simulink model "robot"  (R2018a)
settings: Solver=VariableStepAuto  StartTime=0.0  StopTime=10  RelTol=1e-3
undefined symbols (not defined in the file or in its folder): arm, belt, bread1, bread2
settings Model: Creator=hugo  LastModifiedBy=hugo

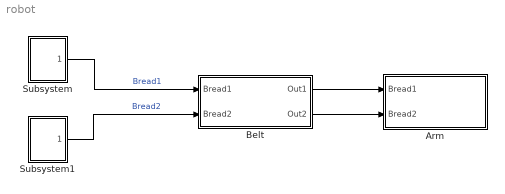
== system robot ==
  Arm : Subsystem
  Belt : Subsystem
  Subsystem : Subsystem
  Subsystem1 : Subsystem
  wires:
  Subsystem/1(Bread1) -> Belt/1(Bread1)  "Bread1"
  Subsystem1/1(Bread2) -> Belt/2(Bread2)  "Bread2"
  Belt/1(Out1) -> Arm/1(Bread1)
  Belt/2(Out2) -> Arm/2(Bread2)

== system robot/Arm ==
  Bread1 : Inport
  Bread2 : Inport  Port=2
  Home Position : Subsystem
  Laser Scanner : Subsystem
  Laser Scanner1 : Subsystem
  MoveArmToBread1 : Subsystem
  MoveArmToBread2 : Subsystem
  MoveArmToHome : Subsystem
  Terminator : Terminator
  To Workspace : ToWorkspace  VariableName=bread1SIM  SaveFormat=Timeseries  SampleTime=-1
  wires:
  Bread1/1 -> To Workspace/1, Laser Scanner/1(In1)
  MoveArmToBread1/1(endEffector) -> MoveArmToBread2/1(Starting Position)
  MoveArmToBread2/1(endEffector) -> MoveArmToHome/1(Starting Position)
  Home Position/1(Home) -> MoveArmToHome/2(Final Position), MoveArmToBread1/1(Starting Position)
  MoveArmToHome/1(endEffector) -> Terminator/1
  Laser Scanner/1(Out1) -> MoveArmToBread1/2(Final Position)
  Bread2/1 -> Laser Scanner1/1(In1)
  Laser Scanner1/1(Out1) -> MoveArmToBread2/2(Final Position)

== system robot/Belt ==
  Bread1 : Inport
  Bread2 : Inport  Port=2
  Constant : Constant  Value=belt.speed
  Movement1 : Subsystem
  Movement2 : Subsystem
  Out1 : Outport
  Out2 : Outport  Port=2
  wires:
  Bread1/1 -> Movement2/2(Bread)
  Movement2/1(Out2) -> Out1/1  "Bread1"
  Movement1/1(Out2) -> Out2/1  "Bread2"
  Bread2/1 -> Movement1/2(Bread)
  Constant/1 -> Movement1/1(Speed), Movement2/1(Speed)

== system robot/Subsystem ==
  Constant : Constant  Value=bread1.x
  Constant1 : Constant  Value=bread1.y
  Constant2 : Constant  Value=bread1.z
  Constant3 : Constant  Value=bread1.theta
  Mux : Mux
  Bread1 : Outport
  wires:
  Mux/1 -> Bread1/1
  Constant/1 -> Mux/1
  Constant1/1 -> Mux/2
  Constant2/1 -> Mux/3
  Constant3/1 -> Mux/4

== system robot/Subsystem1 ==
  Constant : Constant  Value=bread2.x
  Constant1 : Constant  Value=bread2.y
  Constant2 : Constant  Value=bread2.z
  Constant3 : Constant  Value=bread2.theta
  Mux : Mux
  Bread2 : Outport
  wires:
  Mux/1 -> Bread2/1
  Constant/1 -> Mux/1
  Constant1/1 -> Mux/2
  Constant2/1 -> Mux/3
  Constant3/1 -> Mux/4

== system robot/Arm/Home Position ==
  Constant : Constant  Value=arm.homeX
  Constant1 : Constant  Value=arm.homeZ
  Constant2 : Constant  Value=arm.homeY
  Constant3 : Constant  Value=arm.homeZ
  Mux : Mux
  Home : Outport
  wires:
  Constant1/1 -> Mux/3
  Constant2/1 -> Mux/2
  Constant/1 -> Mux/1
  Mux/1 -> Home/1
  Constant3/1 -> Mux/4

== system robot/Arm/Laser Scanner ==
  In1 : Inport
  Demux : Demux
  Mux : Mux
  Switch : Switch  Threshold=0.28
  Out1 : Outport
  wires:
  Switch/1 -> Mux/2
  Demux/4 -> Mux/4  "theta"
  Demux/2 -> Switch/1, Switch/3, Switch/2  "y"
  Demux/1 -> Mux/1  "x"
  Demux/3 -> Mux/3  "z"
  In1/1 -> Demux/1
  Mux/1 -> Out1/1

== system robot/Arm/Laser Scanner1 ==
  In1 : Inport
  Demux : Demux
  Mux : Mux
  Switch : Switch  Threshold=0.28
  Out1 : Outport
  wires:
  Switch/1 -> Mux/2
  Demux/4 -> Mux/4  "theta"
  Demux/2 -> Switch/1, Switch/3, Switch/2  "y"
  Demux/1 -> Mux/1  "x"
  Demux/3 -> Mux/3  "z"
  In1/1 -> Demux/1
  Mux/1 -> Out1/1

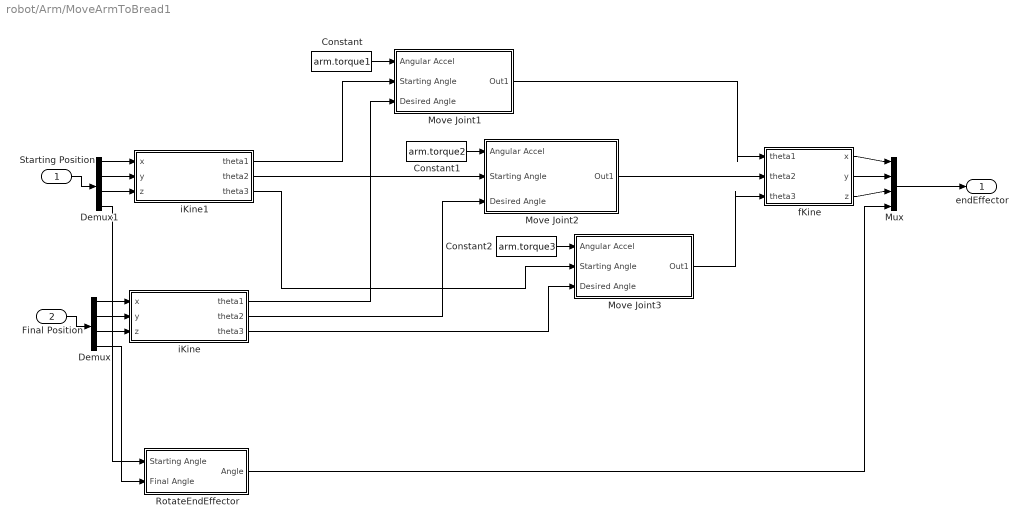
== system robot/Arm/MoveArmToBread1 ==
  Starting Position : Inport
  Final Position : Inport  Port=2
  Constant : Constant  Value=arm.torque1
  Constant1 : Constant  Value=arm.torque2
  Constant2 : Constant  Value=arm.torque3
  Demux : Demux
  Demux1 : Demux
  Move Joint1 : Subsystem
  Move Joint2 : Subsystem
  Move Joint3 : Subsystem
  Mux : Mux
  RotateEndEffector : Subsystem
  fKine : MATLAB Function  TreatAsAtomicUnit=on
  iKine : MATLAB Function  TreatAsAtomicUnit=on
  iKine1 : MATLAB Function  TreatAsAtomicUnit=on
  endEffector : Outport
  wires:
  iKine/1(theta1) -> Move Joint1/3(Desired Angle)
  Starting Position/1 -> Demux1/1
  Demux/2 -> iKine/2(y)
  Demux/3 -> iKine/3(z)
  iKine/2(theta2) -> Move Joint2/3(Desired Angle)
  iKine/3(theta3) -> Move Joint3/3(Desired Angle)
  Move Joint2/1(Out1) -> fKine/2(theta2)
  Move Joint3/1(Out1) -> fKine/3(theta3)
  fKine/1(x) -> Mux/1
  fKine/2(y) -> Mux/2
  fKine/3(z) -> Mux/3
  Mux/1 -> endEffector/1
  Move Joint1/1(Out1) -> fKine/1(theta1)
  Final Position/1 -> Demux/1
  Demux/1 -> iKine/1(x)
  Demux1/2 -> iKine1/2(y)
  Demux1/1 -> iKine1/1(x)
  Demux1/3 -> iKine1/3(z)
  iKine1/1(theta1) -> Move Joint1/2(Starting Angle)
  iKine1/2(theta2) -> Move Joint2/2(Starting Angle)
  iKine1/3(theta3) -> Move Joint3/2(Starting Angle)
  Constant2/1 -> Move Joint3/1(Angular Accel)
  Constant1/1 -> Move Joint2/1(Angular Accel)
  Constant/1 -> Move Joint1/1(Angular Accel)
  Demux1/4 -> RotateEndEffector/1(Starting Angle)
  Demux/4 -> RotateEndEffector/2(Final Angle)
  RotateEndEffector/1(Angle) -> Mux/4

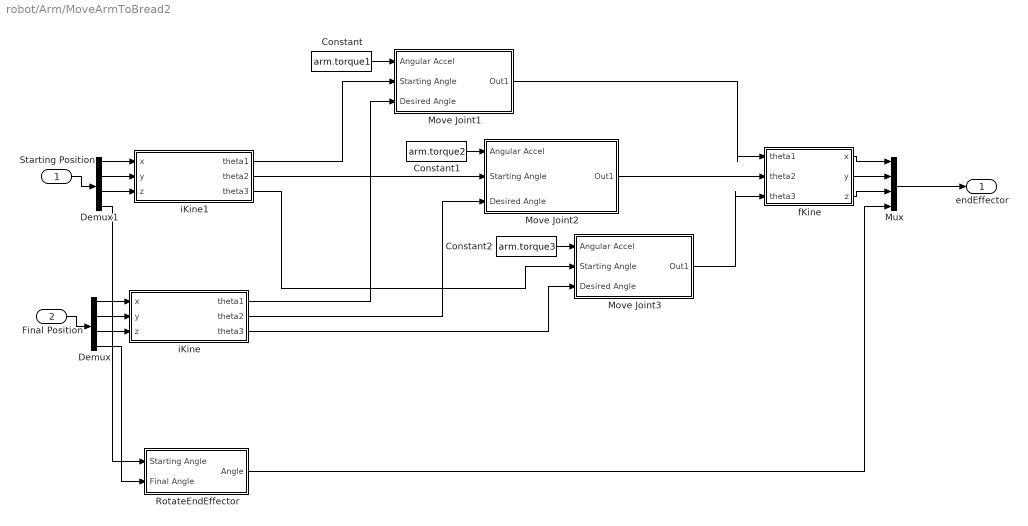
== system robot/Arm/MoveArmToBread2 ==
  Starting Position : Inport
  Final Position : Inport  Port=2
  Constant : Constant  Value=arm.torque1
  Constant1 : Constant  Value=arm.torque2
  Constant2 : Constant  Value=arm.torque3
  Demux : Demux
  Demux1 : Demux
  Move Joint1 : Subsystem
  Move Joint2 : Subsystem
  Move Joint3 : Subsystem
  Mux : Mux
  RotateEndEffector : Subsystem
  fKine : MATLAB Function  TreatAsAtomicUnit=on
  iKine : MATLAB Function  TreatAsAtomicUnit=on
  iKine1 : MATLAB Function  TreatAsAtomicUnit=on
  endEffector : Outport
  wires:
  iKine/1(theta1) -> Move Joint1/3(Desired Angle)
  Starting Position/1 -> Demux1/1
  Demux/2 -> iKine/2(y)
  Demux/3 -> iKine/3(z)
  iKine/2(theta2) -> Move Joint2/3(Desired Angle)
  iKine/3(theta3) -> Move Joint3/3(Desired Angle)
  Move Joint2/1(Out1) -> fKine/2(theta2)
  Move Joint3/1(Out1) -> fKine/3(theta3)
  fKine/1(x) -> Mux/1
  fKine/2(y) -> Mux/2
  fKine/3(z) -> Mux/3
  Mux/1 -> endEffector/1
  Move Joint1/1(Out1) -> fKine/1(theta1)
  Final Position/1 -> Demux/1
  Demux/1 -> iKine/1(x)
  Demux1/2 -> iKine1/2(y)
  Demux1/1 -> iKine1/1(x)
  Demux1/3 -> iKine1/3(z)
  iKine1/1(theta1) -> Move Joint1/2(Starting Angle)
  iKine1/2(theta2) -> Move Joint2/2(Starting Angle)
  iKine1/3(theta3) -> Move Joint3/2(Starting Angle)
  Constant2/1 -> Move Joint3/1(Angular Accel)
  Constant1/1 -> Move Joint2/1(Angular Accel)
  Constant/1 -> Move Joint1/1(Angular Accel)
  Demux1/4 -> RotateEndEffector/1(Starting Angle)
  Demux/4 -> RotateEndEffector/2(Final Angle)
  RotateEndEffector/1(Angle) -> Mux/4

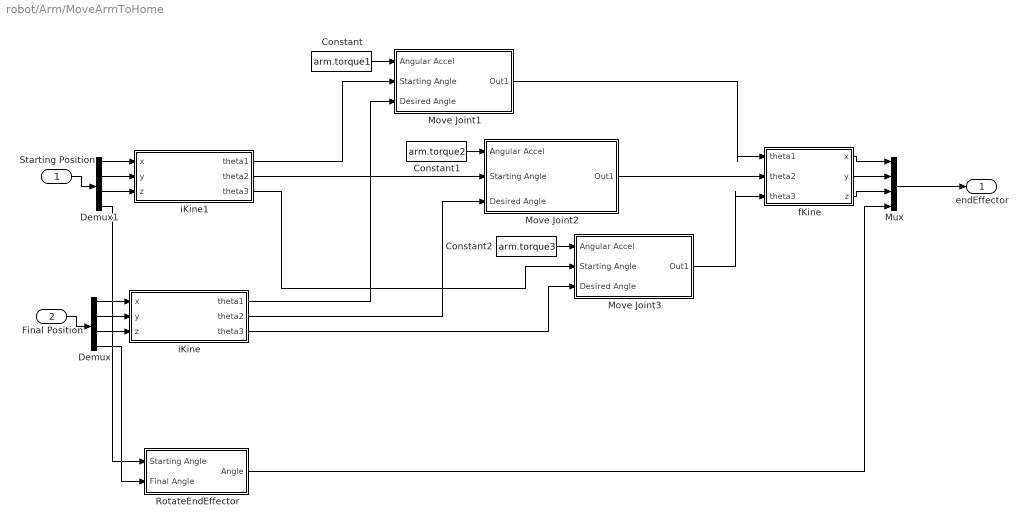
== system robot/Arm/MoveArmToHome ==
  Starting Position : Inport
  Final Position : Inport  Port=2
  Constant : Constant  Value=arm.torque1
  Constant1 : Constant  Value=arm.torque2
  Constant2 : Constant  Value=arm.torque3
  Demux : Demux
  Demux1 : Demux
  Move Joint1 : Subsystem
  Move Joint2 : Subsystem
  Move Joint3 : Subsystem
  Mux : Mux
  RotateEndEffector : Subsystem
  fKine : MATLAB Function  TreatAsAtomicUnit=on
  iKine : MATLAB Function  TreatAsAtomicUnit=on
  iKine1 : MATLAB Function  TreatAsAtomicUnit=on
  endEffector : Outport
  wires:
  iKine/1(theta1) -> Move Joint1/3(Desired Angle)
  Starting Position/1 -> Demux1/1
  Demux/2 -> iKine/2(y)
  Demux/3 -> iKine/3(z)
  iKine/2(theta2) -> Move Joint2/3(Desired Angle)
  iKine/3(theta3) -> Move Joint3/3(Desired Angle)
  Move Joint2/1(Out1) -> fKine/2(theta2)
  Move Joint3/1(Out1) -> fKine/3(theta3)
  fKine/1(x) -> Mux/1
  fKine/2(y) -> Mux/2
  fKine/3(z) -> Mux/3
  Mux/1 -> endEffector/1
  Move Joint1/1(Out1) -> fKine/1(theta1)
  Final Position/1 -> Demux/1
  Demux/1 -> iKine/1(x)
  Demux1/2 -> iKine1/2(y)
  Demux1/1 -> iKine1/1(x)
  Demux1/3 -> iKine1/3(z)
  iKine1/1(theta1) -> Move Joint1/2(Starting Angle)
  iKine1/2(theta2) -> Move Joint2/2(Starting Angle)
  iKine1/3(theta3) -> Move Joint3/2(Starting Angle)
  Constant2/1 -> Move Joint3/1(Angular Accel)
  Constant1/1 -> Move Joint2/1(Angular Accel)
  Constant/1 -> Move Joint1/1(Angular Accel)
  Demux1/4 -> RotateEndEffector/1(Starting Angle)
  Demux/4 -> RotateEndEffector/2(Final Angle)
  RotateEndEffector/1(Angle) -> Mux/4

== system robot/Belt/Movement1 ==
  Speed : Inport
  Bread : Inport  Port=2
  Demux : Demux
  Integrator : Integrator
  Mux : Mux
  Sum : Sum  Inputs=|++
  Out2 : Outport
  wires:
  Bread/1 -> Demux/1  "bread"
  Demux/1 -> Mux/1  "x"
  Demux/3 -> Mux/3  "z"
  Demux/2 -> Sum/2  "y"
  Mux/1 -> Out2/1  "bread.moving"
  Sum/1 -> Mux/2  "y"
  Demux/4 -> Mux/4  "theta"
  Speed/1 -> Integrator/1
  Integrator/1 -> Sum/1

== system robot/Belt/Movement2 ==
  Speed : Inport
  Bread : Inport  Port=2
  Demux : Demux
  Integrator : Integrator
  Mux : Mux
  Sum : Sum  Inputs=|+-
  Out2 : Outport
  wires:
  Bread/1 -> Demux/1  "bread"
  Demux/1 -> Mux/1  "x"
  Demux/3 -> Mux/3  "z"
  Mux/1 -> Out2/1  "bread.moving"
  Sum/1 -> Mux/2  "y"
  Demux/4 -> Mux/4  "theta"
  Speed/1 -> Integrator/1
  Demux/2 -> Sum/1  "y"
  Integrator/1 -> Sum/2

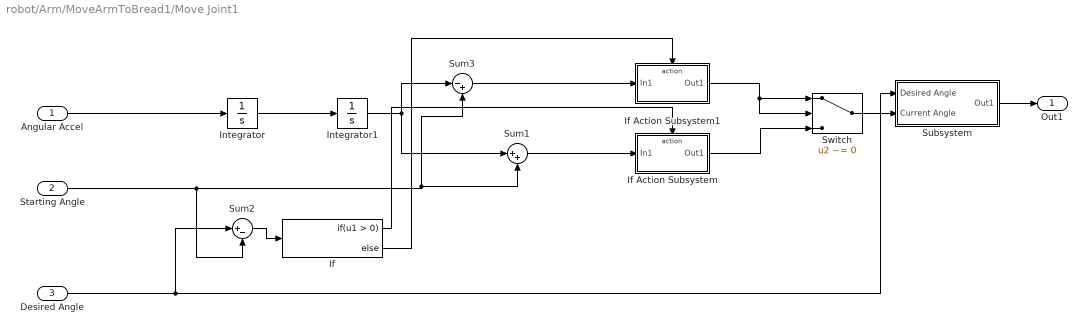
== system robot/Arm/MoveArmToBread1/Move Joint1 ==
  Angular Accel : Inport
  Starting Angle : Inport  Port=2
  Desired Angle : Inport  Port=3
  If : If
  If Action Subsystem : Subsystem  TreatAsAtomicUnit=on
  If Action Subsystem1 : Subsystem  TreatAsAtomicUnit=on
  Integrator : Integrator
  Integrator1 : Integrator
  Subsystem : Subsystem
  Sum1 : Sum  Inputs=|++
  Sum2 : Sum  Inputs=|+-
  Sum3 : Sum  Inputs=|-+
  Switch : Switch  Criteria=u2 ~= 0
  Out1 : Outport
  wires:
  Angular Accel/1 -> Integrator/1
  Integrator/1 -> Integrator1/1
  If Action Subsystem/1(Out1) -> Switch/3
  Sum2/1 -> If/1
  If/2 -> If Action Subsystem1/Action
  Starting Angle/1 -> Sum2/2, Sum3/2, Sum1/2
  Desired Angle/1 -> Subsystem/1(Desired Angle), Sum2/1
  If Action Subsystem1/1(Out1) -> Switch/1, Switch/2
  If/1 -> If Action Subsystem/Action
  Integrator1/1 -> Sum1/1, Sum3/1
  Sum3/1 -> If Action Subsystem1/1(In1)
  Sum1/1 -> If Action Subsystem/1(In1)
  Switch/1 -> Subsystem/2(Current Angle)
  Subsystem/1(Out1) -> Out1/1

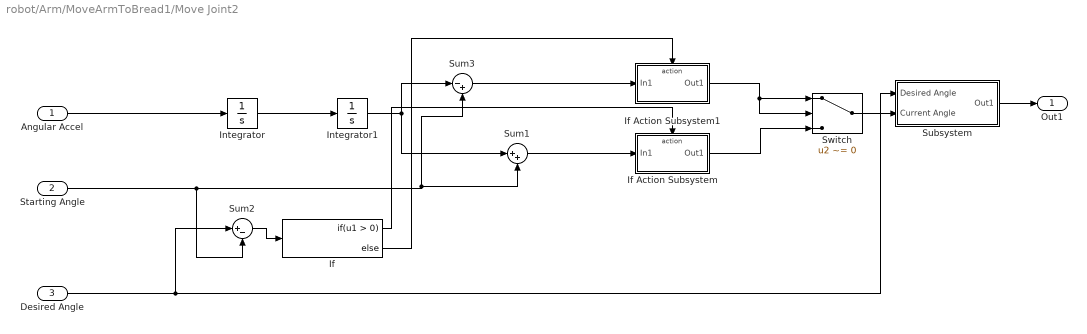
== system robot/Arm/MoveArmToBread1/Move Joint2 ==
  Angular Accel : Inport
  Starting Angle : Inport  Port=2
  Desired Angle : Inport  Port=3
  If : If
  If Action Subsystem : Subsystem  TreatAsAtomicUnit=on
  If Action Subsystem1 : Subsystem  TreatAsAtomicUnit=on
  Integrator : Integrator
  Integrator1 : Integrator
  Subsystem : Subsystem
  Sum1 : Sum  Inputs=|++
  Sum2 : Sum  Inputs=|+-
  Sum3 : Sum  Inputs=|-+
  Switch : Switch  Criteria=u2 ~= 0
  Out1 : Outport
  wires:
  Angular Accel/1 -> Integrator/1
  Integrator/1 -> Integrator1/1
  If Action Subsystem/1(Out1) -> Switch/3
  Sum2/1 -> If/1
  If/2 -> If Action Subsystem1/Action
  Starting Angle/1 -> Sum2/2, Sum3/2, Sum1/2
  Desired Angle/1 -> Subsystem/1(Desired Angle), Sum2/1
  If Action Subsystem1/1(Out1) -> Switch/1, Switch/2
  If/1 -> If Action Subsystem/Action
  Integrator1/1 -> Sum1/1, Sum3/1
  Sum3/1 -> If Action Subsystem1/1(In1)
  Sum1/1 -> If Action Subsystem/1(In1)
  Switch/1 -> Subsystem/2(Current Angle)
  Subsystem/1(Out1) -> Out1/1

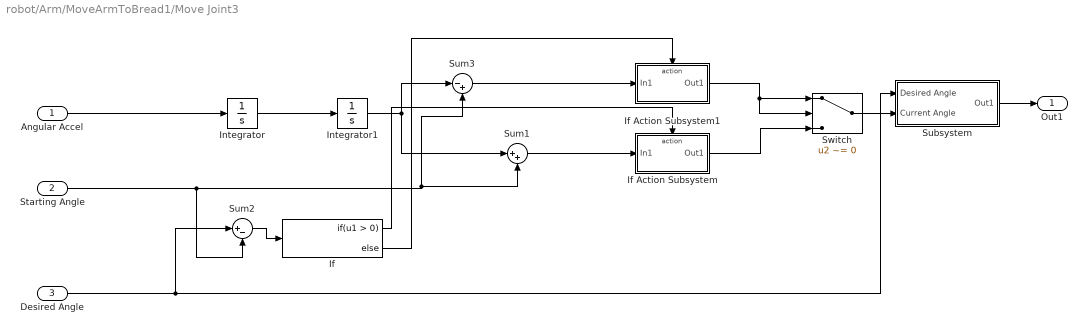
== system robot/Arm/MoveArmToBread1/Move Joint3 ==
  Angular Accel : Inport
  Starting Angle : Inport  Port=2
  Desired Angle : Inport  Port=3
  If : If
  If Action Subsystem : Subsystem  TreatAsAtomicUnit=on
  If Action Subsystem1 : Subsystem  TreatAsAtomicUnit=on
  Integrator : Integrator
  Integrator1 : Integrator
  Subsystem : Subsystem
  Sum1 : Sum  Inputs=|++
  Sum2 : Sum  Inputs=|+-
  Sum3 : Sum  Inputs=|-+
  Switch : Switch  Criteria=u2 ~= 0
  Out1 : Outport
  wires:
  Angular Accel/1 -> Integrator/1
  Integrator/1 -> Integrator1/1
  If Action Subsystem/1(Out1) -> Switch/3
  Sum2/1 -> If/1
  If/2 -> If Action Subsystem1/Action
  Starting Angle/1 -> Sum2/2, Sum3/2, Sum1/2
  Desired Angle/1 -> Subsystem/1(Desired Angle), Sum2/1
  If Action Subsystem1/1(Out1) -> Switch/1, Switch/2
  If/1 -> If Action Subsystem/Action
  Integrator1/1 -> Sum1/1, Sum3/1
  Sum3/1 -> If Action Subsystem1/1(In1)
  Sum1/1 -> If Action Subsystem/1(In1)
  Switch/1 -> Subsystem/2(Current Angle)
  Subsystem/1(Out1) -> Out1/1

== system robot/Arm/MoveArmToBread1/RotateEndEffector ==
  Starting Angle : Inport
  Final Angle : Inport  Port=2
  Terminator : Terminator
  Angle : Outport
  wires:
  Final Angle/1 -> Angle/1
  Starting Angle/1 -> Terminator/1

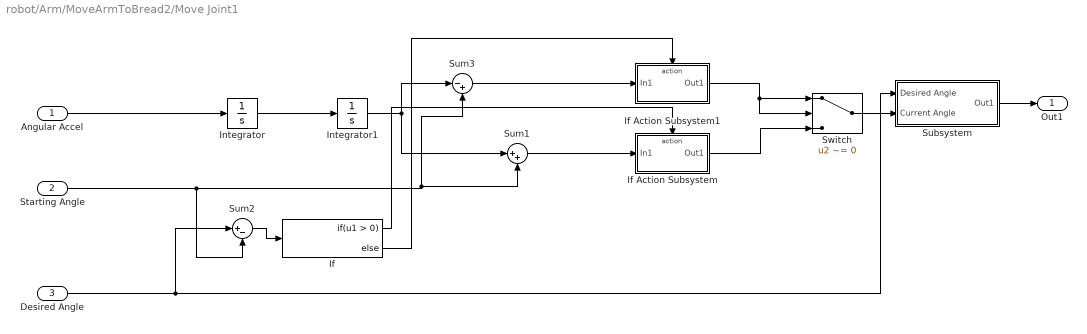
== system robot/Arm/MoveArmToBread2/Move Joint1 ==
  Angular Accel : Inport
  Starting Angle : Inport  Port=2
  Desired Angle : Inport  Port=3
  If : If
  If Action Subsystem : Subsystem  TreatAsAtomicUnit=on
  If Action Subsystem1 : Subsystem  TreatAsAtomicUnit=on
  Integrator : Integrator
  Integrator1 : Integrator
  Subsystem : Subsystem
  Sum1 : Sum  Inputs=|++
  Sum2 : Sum  Inputs=|+-
  Sum3 : Sum  Inputs=|-+
  Switch : Switch  Criteria=u2 ~= 0
  Out1 : Outport
  wires:
  Angular Accel/1 -> Integrator/1
  Integrator/1 -> Integrator1/1
  If Action Subsystem/1(Out1) -> Switch/3
  Sum2/1 -> If/1
  If/2 -> If Action Subsystem1/Action
  Starting Angle/1 -> Sum2/2, Sum3/2, Sum1/2
  Desired Angle/1 -> Subsystem/1(Desired Angle), Sum2/1
  If Action Subsystem1/1(Out1) -> Switch/1, Switch/2
  If/1 -> If Action Subsystem/Action
  Integrator1/1 -> Sum1/1, Sum3/1
  Sum3/1 -> If Action Subsystem1/1(In1)
  Sum1/1 -> If Action Subsystem/1(In1)
  Switch/1 -> Subsystem/2(Current Angle)
  Subsystem/1(Out1) -> Out1/1

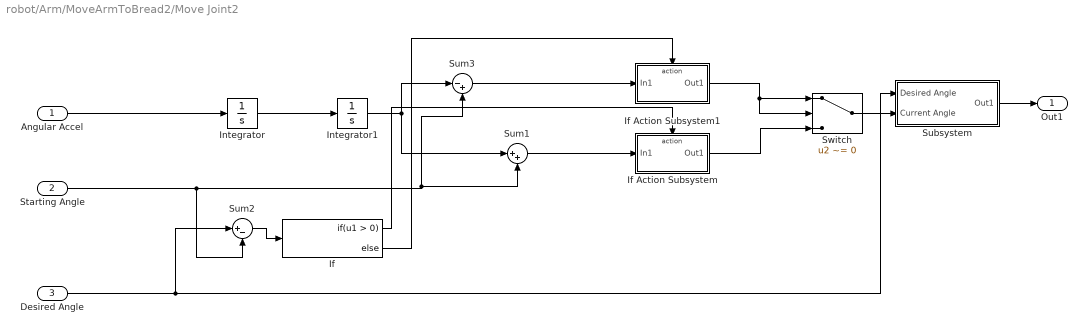
== system robot/Arm/MoveArmToBread2/Move Joint2 ==
  Angular Accel : Inport
  Starting Angle : Inport  Port=2
  Desired Angle : Inport  Port=3
  If : If
  If Action Subsystem : Subsystem  TreatAsAtomicUnit=on
  If Action Subsystem1 : Subsystem  TreatAsAtomicUnit=on
  Integrator : Integrator
  Integrator1 : Integrator
  Subsystem : Subsystem
  Sum1 : Sum  Inputs=|++
  Sum2 : Sum  Inputs=|+-
  Sum3 : Sum  Inputs=|-+
  Switch : Switch  Criteria=u2 ~= 0
  Out1 : Outport
  wires:
  Angular Accel/1 -> Integrator/1
  Integrator/1 -> Integrator1/1
  If Action Subsystem/1(Out1) -> Switch/3
  Sum2/1 -> If/1
  If/2 -> If Action Subsystem1/Action
  Starting Angle/1 -> Sum2/2, Sum3/2, Sum1/2
  Desired Angle/1 -> Subsystem/1(Desired Angle), Sum2/1
  If Action Subsystem1/1(Out1) -> Switch/1, Switch/2
  If/1 -> If Action Subsystem/Action
  Integrator1/1 -> Sum1/1, Sum3/1
  Sum3/1 -> If Action Subsystem1/1(In1)
  Sum1/1 -> If Action Subsystem/1(In1)
  Switch/1 -> Subsystem/2(Current Angle)
  Subsystem/1(Out1) -> Out1/1

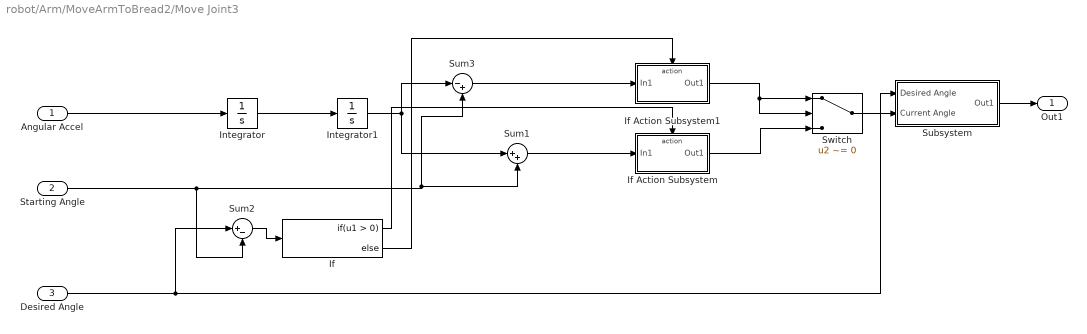
== system robot/Arm/MoveArmToBread2/Move Joint3 ==
  Angular Accel : Inport
  Starting Angle : Inport  Port=2
  Desired Angle : Inport  Port=3
  If : If
  If Action Subsystem : Subsystem  TreatAsAtomicUnit=on
  If Action Subsystem1 : Subsystem  TreatAsAtomicUnit=on
  Integrator : Integrator
  Integrator1 : Integrator
  Subsystem : Subsystem
  Sum1 : Sum  Inputs=|++
  Sum2 : Sum  Inputs=|+-
  Sum3 : Sum  Inputs=|-+
  Switch : Switch  Criteria=u2 ~= 0
  Out1 : Outport
  wires:
  Angular Accel/1 -> Integrator/1
  Integrator/1 -> Integrator1/1
  If Action Subsystem/1(Out1) -> Switch/3
  Sum2/1 -> If/1
  If/2 -> If Action Subsystem1/Action
  Starting Angle/1 -> Sum2/2, Sum3/2, Sum1/2
  Desired Angle/1 -> Subsystem/1(Desired Angle), Sum2/1
  If Action Subsystem1/1(Out1) -> Switch/1, Switch/2
  If/1 -> If Action Subsystem/Action
  Integrator1/1 -> Sum1/1, Sum3/1
  Sum3/1 -> If Action Subsystem1/1(In1)
  Sum1/1 -> If Action Subsystem/1(In1)
  Switch/1 -> Subsystem/2(Current Angle)
  Subsystem/1(Out1) -> Out1/1

== system robot/Arm/MoveArmToBread2/RotateEndEffector ==
  Starting Angle : Inport
  Final Angle : Inport  Port=2
  Terminator : Terminator
  Angle : Outport
  wires:
  Final Angle/1 -> Angle/1
  Starting Angle/1 -> Terminator/1

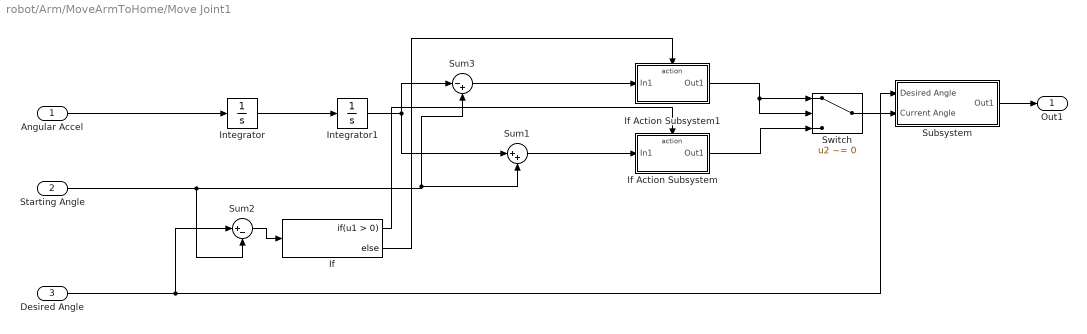
== system robot/Arm/MoveArmToHome/Move Joint1 ==
  Angular Accel : Inport
  Starting Angle : Inport  Port=2
  Desired Angle : Inport  Port=3
  If : If
  If Action Subsystem : Subsystem  TreatAsAtomicUnit=on
  If Action Subsystem1 : Subsystem  TreatAsAtomicUnit=on
  Integrator : Integrator
  Integrator1 : Integrator
  Subsystem : Subsystem
  Sum1 : Sum  Inputs=|++
  Sum2 : Sum  Inputs=|+-
  Sum3 : Sum  Inputs=|-+
  Switch : Switch  Criteria=u2 ~= 0
  Out1 : Outport
  wires:
  Angular Accel/1 -> Integrator/1
  Integrator/1 -> Integrator1/1
  If Action Subsystem/1(Out1) -> Switch/3
  Sum2/1 -> If/1
  If/2 -> If Action Subsystem1/Action
  Starting Angle/1 -> Sum2/2, Sum3/2, Sum1/2
  Desired Angle/1 -> Subsystem/1(Desired Angle), Sum2/1
  If Action Subsystem1/1(Out1) -> Switch/1, Switch/2
  If/1 -> If Action Subsystem/Action
  Integrator1/1 -> Sum1/1, Sum3/1
  Sum3/1 -> If Action Subsystem1/1(In1)
  Sum1/1 -> If Action Subsystem/1(In1)
  Switch/1 -> Subsystem/2(Current Angle)
  Subsystem/1(Out1) -> Out1/1

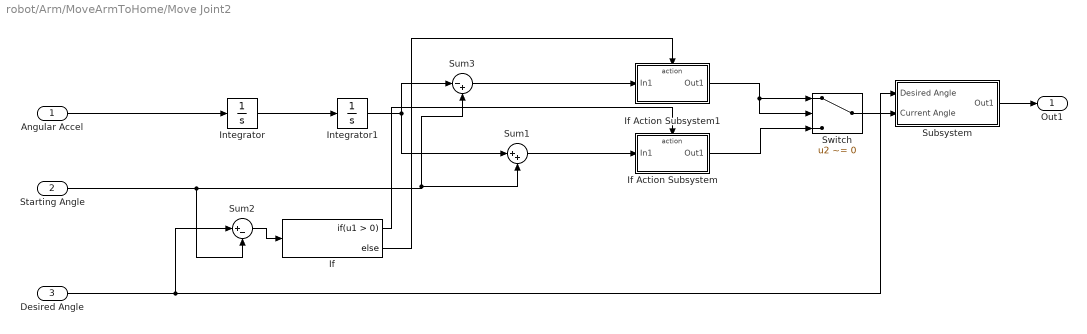
== system robot/Arm/MoveArmToHome/Move Joint2 ==
  Angular Accel : Inport
  Starting Angle : Inport  Port=2
  Desired Angle : Inport  Port=3
  If : If
  If Action Subsystem : Subsystem  TreatAsAtomicUnit=on
  If Action Subsystem1 : Subsystem  TreatAsAtomicUnit=on
  Integrator : Integrator
  Integrator1 : Integrator
  Subsystem : Subsystem
  Sum1 : Sum  Inputs=|++
  Sum2 : Sum  Inputs=|+-
  Sum3 : Sum  Inputs=|-+
  Switch : Switch  Criteria=u2 ~= 0
  Out1 : Outport
  wires:
  Angular Accel/1 -> Integrator/1
  Integrator/1 -> Integrator1/1
  If Action Subsystem/1(Out1) -> Switch/3
  Sum2/1 -> If/1
  If/2 -> If Action Subsystem1/Action
  Starting Angle/1 -> Sum2/2, Sum3/2, Sum1/2
  Desired Angle/1 -> Subsystem/1(Desired Angle), Sum2/1
  If Action Subsystem1/1(Out1) -> Switch/1, Switch/2
  If/1 -> If Action Subsystem/Action
  Integrator1/1 -> Sum1/1, Sum3/1
  Sum3/1 -> If Action Subsystem1/1(In1)
  Sum1/1 -> If Action Subsystem/1(In1)
  Switch/1 -> Subsystem/2(Current Angle)
  Subsystem/1(Out1) -> Out1/1

== system robot/Arm/MoveArmToHome/Move Joint3 ==
  Angular Accel : Inport
  Starting Angle : Inport  Port=2
  Desired Angle : Inport  Port=3
  If : If
  If Action Subsystem : Subsystem  TreatAsAtomicUnit=on
  If Action Subsystem1 : Subsystem  TreatAsAtomicUnit=on
  Integrator : Integrator
  Integrator1 : Integrator
  Subsystem : Subsystem
  Sum1 : Sum  Inputs=|++
  Sum2 : Sum  Inputs=|+-
  Sum3 : Sum  Inputs=|-+
  Switch : Switch  Criteria=u2 ~= 0
  Out1 : Outport
  wires:
  Angular Accel/1 -> Integrator/1
  Integrator/1 -> Integrator1/1
  If Action Subsystem/1(Out1) -> Switch/3
  Sum2/1 -> If/1
  If/2 -> If Action Subsystem1/Action
  Starting Angle/1 -> Sum2/2, Sum3/2, Sum1/2
  Desired Angle/1 -> Subsystem/1(Desired Angle), Sum2/1
  If Action Subsystem1/1(Out1) -> Switch/1, Switch/2
  If/1 -> If Action Subsystem/Action
  Integrator1/1 -> Sum1/1, Sum3/1
  Sum3/1 -> If Action Subsystem1/1(In1)
  Sum1/1 -> If Action Subsystem/1(In1)
  Switch/1 -> Subsystem/2(Current Angle)
  Subsystem/1(Out1) -> Out1/1

== system robot/Arm/MoveArmToHome/RotateEndEffector ==
  Starting Angle : Inport
  Final Angle : Inport  Port=2
  Terminator : Terminator
  Angle : Outport
  wires:
  Final Angle/1 -> Angle/1
  Starting Angle/1 -> Terminator/1

== system robot/Arm/MoveArmToBread1/Move Joint1/If Action Subsystem ==
  In1 : Inport
  Action Port : ActionPort  ActionType=then
  Out1 : Outport
  wires:
  In1/1 -> Out1/1

== system robot/Arm/MoveArmToBread1/Move Joint1/If Action Subsystem1 ==
  In1 : Inport
  Action Port : ActionPort  ActionType=else
  Out1 : Outport
  wires:
  In1/1 -> Out1/1

== system robot/Arm/MoveArmToBread1/Move Joint1/Subsystem ==
  Desired Angle : Inport
  Current Angle : Inport  Port=2
  Abs : Abs
  Constant : Constant  Value=0.1
  Logical Operator : Logic  Operator=OR  AllPortsSameDT=off  OutDataTypeStr=boolean
  Memory : Memory
  Relational Operator : RelationalOperator  Operator=<=  OutDataTypeStr=boolean  RndMeth=Simplest
  Sum : Sum  Inputs=|+-
  Switch1 : Switch  Criteria=u2 > Threshold
  Out1 : Outport
  wires:
  Switch1/1 -> Out1/1
  Desired Angle/1 -> Sum/1, Switch1/1
  Current Angle/1 -> Switch1/3, Sum/2
  Sum/1 -> Abs/1
  Abs/1 -> Relational Operator/1
  Constant/1 -> Relational Operator/2
  Relational Operator/1 -> Logical Operator/2
  Logical Operator/1 -> Memory/1, Switch1/2
  Memory/1 -> Logical Operator/1

== system robot/Arm/MoveArmToBread1/Move Joint2/If Action Subsystem ==
  In1 : Inport
  Action Port : ActionPort  ActionType=then
  Out1 : Outport
  wires:
  In1/1 -> Out1/1

== system robot/Arm/MoveArmToBread1/Move Joint2/If Action Subsystem1 ==
  In1 : Inport
  Action Port : ActionPort  ActionType=else
  Out1 : Outport
  wires:
  In1/1 -> Out1/1

== system robot/Arm/MoveArmToBread1/Move Joint2/Subsystem ==
  Desired Angle : Inport
  Current Angle : Inport  Port=2
  Abs : Abs
  Constant : Constant  Value=0.1
  Logical Operator : Logic  Operator=OR  AllPortsSameDT=off  OutDataTypeStr=boolean
  Memory : Memory
  Relational Operator : RelationalOperator  Operator=<=  OutDataTypeStr=boolean  RndMeth=Simplest
  Sum : Sum  Inputs=|+-
  Switch1 : Switch  Criteria=u2 > Threshold
  Out1 : Outport
  wires:
  Switch1/1 -> Out1/1
  Desired Angle/1 -> Sum/1, Switch1/1
  Current Angle/1 -> Switch1/3, Sum/2
  Sum/1 -> Abs/1
  Abs/1 -> Relational Operator/1
  Constant/1 -> Relational Operator/2
  Relational Operator/1 -> Logical Operator/2
  Logical Operator/1 -> Memory/1, Switch1/2
  Memory/1 -> Logical Operator/1

== system robot/Arm/MoveArmToBread1/Move Joint3/If Action Subsystem ==
  In1 : Inport
  Action Port : ActionPort  ActionType=then
  Out1 : Outport
  wires:
  In1/1 -> Out1/1

== system robot/Arm/MoveArmToBread1/Move Joint3/If Action Subsystem1 ==
  In1 : Inport
  Action Port : ActionPort  ActionType=else
  Out1 : Outport
  wires:
  In1/1 -> Out1/1

== system robot/Arm/MoveArmToBread1/Move Joint3/Subsystem ==
  Desired Angle : Inport
  Current Angle : Inport  Port=2
  Abs : Abs
  Constant : Constant  Value=0.1
  Logical Operator : Logic  Operator=OR  AllPortsSameDT=off  OutDataTypeStr=boolean
  Memory : Memory
  Relational Operator : RelationalOperator  Operator=<=  OutDataTypeStr=boolean  RndMeth=Simplest
  Sum : Sum  Inputs=|+-
  Switch1 : Switch  Criteria=u2 > Threshold
  Out1 : Outport
  wires:
  Switch1/1 -> Out1/1
  Desired Angle/1 -> Sum/1, Switch1/1
  Current Angle/1 -> Switch1/3, Sum/2
  Sum/1 -> Abs/1
  Abs/1 -> Relational Operator/1
  Constant/1 -> Relational Operator/2
  Relational Operator/1 -> Logical Operator/2
  Logical Operator/1 -> Memory/1, Switch1/2
  Memory/1 -> Logical Operator/1

== system robot/Arm/MoveArmToBread2/Move Joint1/If Action Subsystem ==
  In1 : Inport
  Action Port : ActionPort  ActionType=then
  Out1 : Outport
  wires:
  In1/1 -> Out1/1

== system robot/Arm/MoveArmToBread2/Move Joint1/If Action Subsystem1 ==
  In1 : Inport
  Action Port : ActionPort  ActionType=else
  Out1 : Outport
  wires:
  In1/1 -> Out1/1

== system robot/Arm/MoveArmToBread2/Move Joint1/Subsystem ==
  Desired Angle : Inport
  Current Angle : Inport  Port=2
  Abs : Abs
  Constant : Constant  Value=0.1
  Logical Operator : Logic  Operator=OR  AllPortsSameDT=off  OutDataTypeStr=boolean
  Memory : Memory
  Relational Operator : RelationalOperator  Operator=<=  OutDataTypeStr=boolean  RndMeth=Simplest
  Sum : Sum  Inputs=|+-
  Switch1 : Switch  Criteria=u2 > Threshold
  Out1 : Outport
  wires:
  Switch1/1 -> Out1/1
  Desired Angle/1 -> Sum/1, Switch1/1
  Current Angle/1 -> Switch1/3, Sum/2
  Sum/1 -> Abs/1
  Abs/1 -> Relational Operator/1
  Constant/1 -> Relational Operator/2
  Relational Operator/1 -> Logical Operator/2
  Logical Operator/1 -> Memory/1, Switch1/2
  Memory/1 -> Logical Operator/1

== system robot/Arm/MoveArmToBread2/Move Joint2/If Action Subsystem ==
  In1 : Inport
  Action Port : ActionPort  ActionType=then
  Out1 : Outport
  wires:
  In1/1 -> Out1/1

== system robot/Arm/MoveArmToBread2/Move Joint2/If Action Subsystem1 ==
  In1 : Inport
  Action Port : ActionPort  ActionType=else
  Out1 : Outport
  wires:
  In1/1 -> Out1/1

== system robot/Arm/MoveArmToBread2/Move Joint2/Subsystem ==
  Desired Angle : Inport
  Current Angle : Inport  Port=2
  Abs : Abs
  Constant : Constant  Value=0.1
  Logical Operator : Logic  Operator=OR  AllPortsSameDT=off  OutDataTypeStr=boolean
  Memory : Memory
  Relational Operator : RelationalOperator  Operator=<=  OutDataTypeStr=boolean  RndMeth=Simplest
  Sum : Sum  Inputs=|+-
  Switch1 : Switch  Criteria=u2 > Threshold
  Out1 : Outport
  wires:
  Switch1/1 -> Out1/1
  Desired Angle/1 -> Sum/1, Switch1/1
  Current Angle/1 -> Switch1/3, Sum/2
  Sum/1 -> Abs/1
  Abs/1 -> Relational Operator/1
  Constant/1 -> Relational Operator/2
  Relational Operator/1 -> Logical Operator/2
  Logical Operator/1 -> Memory/1, Switch1/2
  Memory/1 -> Logical Operator/1

== system robot/Arm/MoveArmToBread2/Move Joint3/If Action Subsystem ==
  In1 : Inport
  Action Port : ActionPort  ActionType=then
  Out1 : Outport
  wires:
  In1/1 -> Out1/1

== system robot/Arm/MoveArmToBread2/Move Joint3/If Action Subsystem1 ==
  In1 : Inport
  Action Port : ActionPort  ActionType=else
  Out1 : Outport
  wires:
  In1/1 -> Out1/1

== system robot/Arm/MoveArmToBread2/Move Joint3/Subsystem ==
  Desired Angle : Inport
  Current Angle : Inport  Port=2
  Abs : Abs
  Constant : Constant  Value=0.1
  Logical Operator : Logic  Operator=OR  AllPortsSameDT=off  OutDataTypeStr=boolean
  Memory : Memory
  Relational Operator : RelationalOperator  Operator=<=  OutDataTypeStr=boolean  RndMeth=Simplest
  Sum : Sum  Inputs=|+-
  Switch1 : Switch  Criteria=u2 > Threshold
  Out1 : Outport
  wires:
  Switch1/1 -> Out1/1
  Desired Angle/1 -> Sum/1, Switch1/1
  Current Angle/1 -> Switch1/3, Sum/2
  Sum/1 -> Abs/1
  Abs/1 -> Relational Operator/1
  Constant/1 -> Relational Operator/2
  Relational Operator/1 -> Logical Operator/2
  Logical Operator/1 -> Memory/1, Switch1/2
  Memory/1 -> Logical Operator/1

== system robot/Arm/MoveArmToHome/Move Joint1/If Action Subsystem ==
  In1 : Inport
  Action Port : ActionPort  ActionType=then
  Out1 : Outport
  wires:
  In1/1 -> Out1/1

== system robot/Arm/MoveArmToHome/Move Joint1/If Action Subsystem1 ==
  In1 : Inport
  Action Port : ActionPort  ActionType=else
  Out1 : Outport
  wires:
  In1/1 -> Out1/1

== system robot/Arm/MoveArmToHome/Move Joint1/Subsystem ==
  Desired Angle : Inport
  Current Angle : Inport  Port=2
  Abs : Abs
  Constant : Constant  Value=0.1
  Logical Operator : Logic  Operator=OR  AllPortsSameDT=off  OutDataTypeStr=boolean
  Memory : Memory
  Relational Operator : RelationalOperator  Operator=<=  OutDataTypeStr=boolean  RndMeth=Simplest
  Sum : Sum  Inputs=|+-
  Switch1 : Switch  Criteria=u2 > Threshold
  Out1 : Outport
  wires:
  Switch1/1 -> Out1/1
  Desired Angle/1 -> Sum/1, Switch1/1
  Current Angle/1 -> Switch1/3, Sum/2
  Sum/1 -> Abs/1
  Abs/1 -> Relational Operator/1
  Constant/1 -> Relational Operator/2
  Relational Operator/1 -> Logical Operator/2
  Logical Operator/1 -> Memory/1, Switch1/2
  Memory/1 -> Logical Operator/1

== system robot/Arm/MoveArmToHome/Move Joint2/If Action Subsystem ==
  In1 : Inport
  Action Port : ActionPort  ActionType=then
  Out1 : Outport
  wires:
  In1/1 -> Out1/1

== system robot/Arm/MoveArmToHome/Move Joint2/If Action Subsystem1 ==
  In1 : Inport
  Action Port : ActionPort  ActionType=else
  Out1 : Outport
  wires:
  In1/1 -> Out1/1

== system robot/Arm/MoveArmToHome/Move Joint2/Subsystem ==
  Desired Angle : Inport
  Current Angle : Inport  Port=2
  Abs : Abs
  Constant : Constant  Value=0.1
  Logical Operator : Logic  Operator=OR  AllPortsSameDT=off  OutDataTypeStr=boolean
  Memory : Memory
  Relational Operator : RelationalOperator  Operator=<=  OutDataTypeStr=boolean  RndMeth=Simplest
  Sum : Sum  Inputs=|+-
  Switch1 : Switch  Criteria=u2 > Threshold
  Out1 : Outport
  wires:
  Switch1/1 -> Out1/1
  Desired Angle/1 -> Sum/1, Switch1/1
  Current Angle/1 -> Switch1/3, Sum/2
  Sum/1 -> Abs/1
  Abs/1 -> Relational Operator/1
  Constant/1 -> Relational Operator/2
  Relational Operator/1 -> Logical Operator/2
  Logical Operator/1 -> Memory/1, Switch1/2
  Memory/1 -> Logical Operator/1

== system robot/Arm/MoveArmToHome/Move Joint3/If Action Subsystem ==
  In1 : Inport
  Action Port : ActionPort  ActionType=then
  Out1 : Outport
  wires:
  In1/1 -> Out1/1

== system robot/Arm/MoveArmToHome/Move Joint3/If Action Subsystem1 ==
  In1 : Inport
  Action Port : ActionPort  ActionType=else
  Out1 : Outport
  wires:
  In1/1 -> Out1/1

== system robot/Arm/MoveArmToHome/Move Joint3/Subsystem ==
  Desired Angle : Inport
  Current Angle : Inport  Port=2
  Abs : Abs
  Constant : Constant  Value=0.1
  Logical Operator : Logic  Operator=OR  AllPortsSameDT=off  OutDataTypeStr=boolean
  Memory : Memory
  Relational Operator : RelationalOperator  Operator=<=  OutDataTypeStr=boolean  RndMeth=Simplest
  Sum : Sum  Inputs=|+-
  Switch1 : Switch  Criteria=u2 > Threshold
  Out1 : Outport
  wires:
  Switch1/1 -> Out1/1
  Desired Angle/1 -> Sum/1, Switch1/1
  Current Angle/1 -> Switch1/3, Sum/2
  Sum/1 -> Abs/1
  Abs/1 -> Relational Operator/1
  Constant/1 -> Relational Operator/2
  Relational Operator/1 -> Logical Operator/2
  Logical Operator/1 -> Memory/1, Switch1/2
  Memory/1 -> Logical Operator/1

== matlab function robot/Arm/MoveArmToBread1/iKine ==
  data: x input; theta1 output; y input; z input; theta2 output; theta3 output
function [theta1,theta2,theta3] = iKine(x, y, z) 
    theta1 = acos(x/sqrt(x^2 + y^2));
    theta2 = sqrt(x^2 + y^2) - 0.32;
    theta3 = 0.735 - z;
end

== matlab function robot/Arm/MoveArmToBread1/fKine ==
  data: x output; theta1 input; y output; theta2 input; theta3 input; z output
function [x,y,z] = fKine(theta1, theta2, theta3) 
    x = cos(theta1)*(theta2 + 0.32);
    y = sin(theta1)*(theta2 + 0.32);
    z = 0.735 - theta3;
end

== matlab function robot/Arm/MoveArmToBread2/fKine ==
  data: x output; theta1 input; y output; theta2 input; theta3 input; z output
function [x,y,z] = fKine(theta1, theta2, theta3) 
    x = cos(theta1)*(theta2 + 0.32);
    y = sin(theta1)*(theta2 + 0.32);
    z = 0.735 - theta3;
end

== matlab function robot/Arm/MoveArmToBread2/iKine ==
  data: x input; theta1 output; y input; z input; theta2 output; theta3 output
function [theta1,theta2,theta3] = iKine(x, y, z) 
    theta1 = acos(x/sqrt(x^2 + y^2));
    theta2 = sqrt(x^2 + y^2) - 0.32;
    theta3 = 0.735 - z;
end

== matlab function robot/Arm/MoveArmToBread1/iKine1 ==
  data: x input; theta1 output; y input; z input; theta2 output; theta3 output
function [theta1,theta2,theta3] = iKine(x, y, z) 
    theta1 = acos(x/sqrt(x^2 + y^2));
    theta2 = sqrt(x^2 + y^2) - 0.32;
    theta3 = 0.735 - z;
end

== matlab function robot/Arm/MoveArmToBread2/iKine1 ==
  data: x input; theta1 output; y input; z input; theta2 output; theta3 output
function [theta1,theta2,theta3] = iKine(x, y, z) 
    theta1 = acos(x/sqrt(x^2 + y^2));
    theta2 = sqrt(x^2 + y^2) - 0.32;
    theta3 = 0.735 - z;
end

== matlab function robot/Arm/MoveArmToHome/fKine ==
  data: x output; theta1 input; y output; theta2 input; theta3 input; z output
function [x,y,z] = fKine(theta1, theta2, theta3) 
    x = cos(theta1)*(theta2 + 0.32);
    y = sin(theta1)*(theta2 + 0.32);
    z = 0.735 - theta3;
end

== matlab function robot/Arm/MoveArmToHome/iKine ==
  data: x input; theta1 output; y input; z input; theta2 output; theta3 output
function [theta1,theta2,theta3] = iKine(x, y, z) 
    theta1 = acos(x/sqrt(x^2 + y^2));
    theta2 = sqrt(x^2 + y^2) - 0.32;
    theta3 = 0.735 - z;
end

== matlab function robot/Arm/MoveArmToHome/iKine1 ==
  data: x input; theta1 output; y input; z input; theta2 output; theta3 output
function [theta1,theta2,theta3] = iKine(x, y, z) 
    theta1 = acos(x/sqrt(x^2 + y^2));
    theta2 = sqrt(x^2 + y^2) - 0.32;
    theta3 = 0.735 - z;
end
